simulink model "PID_Controller_xynew_2018"  (R2018b)
settings: Solver=ode4  StartTime=0.0  StopTime=50  FixedStep=0.01  RelTol=1e-5
InitFcn:
  | % load parameters of the default quadrotor
  | disp('Quadrotor parameters loaded by InitFcn')
  | mdl_quadrotor
undefined symbols (not defined in the file or in its folder): A, B, C, D, pwm, quad
libraries: vrlib x3, realtime_pacer_lib x2, simulink x1
(part 3 of 4)

== system PID_Controller_xynew_2018/Linear Controller/Position_controller/Subsystem1 ==
  a[0] : Inport
  a[1] : Inport  Port=2
  sin(yaw) : Inport  Port=3
  cos(yaw) : Inport  Port=4
  Gain : Gain  Gain=1/9.81
  Product : Product
  Product1 : Product
  Sum1 : Sum
  Pitch adjust : Outport
  wires:
  Sum1/1 -> Gain/1
  a[0]/1 -> Product/1
  Product/1 -> Sum1/1
  cos(yaw)/1 -> Product/2
  a[1]/1 -> Product1/1
  Product1/1 -> Sum1/2
  Gain/1 -> Pitch adjust/1
  sin(yaw)/1 -> Product1/2

== system PID_Controller_xynew_2018/Linear Controller/Position_controller/pitch controller ==
  x double dot : Inport
  y double dot : Inport  Port=2
  sin(yaw) : Inport  Port=3
  cos(yaw) : Inport  Port=4
  Fcn : Fcn  Expr=1/(u)
  Gain : Gain  Gain=1/9.81
  Product : Product
  Product1 : Product
  Product2 : Product
  Square : Math  Operator=square  SaturateOnIntegerOverflow=on
  Square1 : Math  Operator=square  SaturateOnIntegerOverflow=on
  Sum : Sum  Inputs=|-+
  Sum1 : Sum  Inputs=+-
  Roll adjust : Outport
  wires:
  Square/1 -> Sum/1
  Product1/1 -> Sum1/2
  sin(yaw)/1 -> Square1/1, Product/2
  Product2/1 -> Roll adjust/1
  cos(yaw)/1 -> Square/1, Product1/2
  Sum1/1 -> Gain/1
  x double dot/1 -> Product/1
  Product/1 -> Sum1/1
  Fcn/1 -> Product2/2
  Square1/1 -> Sum/2
  Gain/1 -> Product2/1
  Sum/1 -> Fcn/1
  y double dot/1 -> Product1/1

== system PID_Controller_xynew_2018/Linear Controller/Position_controller1/PID_Roll_Rate2 ==
  Setpoint : Inport
  Measured : Inport  Port=2
  Derivative : Derivative
  Integrator Limited : Integrator  LimitOutput=on  UpperSaturationLimit=0.1  LowerSaturationLimit=-0.1
  Kd : Gain  Gain=0  OutMin=[-200]  OutMax=[200]
  Ki : Gain  Gain=2  OutMin=[-200]  OutMax=[200]
  Kp : Gain  Gain=30  OutMin=[-200]  OutMax=[200]
  Scope : Scope
  Sum5 : Sum  Inputs=+++
  Sum6 : Sum  Inputs=+-|
  Adjust : Outport  VectorParamsAs1DForOutWhenUnconnected=on
  wires:
  Measured/1 -> Sum6/2  "measured"
  Setpoint/1 -> Sum6/1  "pid_desired"
  Ki/1 -> Sum5/2
  Sum5/1 -> Adjust/1
  Kp/1 -> Sum5/1
  Kd/1 -> Sum5/3
  Sum6/1 -> Derivative/1, Integrator Limited/1, Kp/1  "pid_error"
  Integrator Limited/1 -> Scope/1, Ki/1
  Derivative/1 -> Kd/1

== system PID_Controller_xynew_2018/Linear Controller/Position_controller1/PID_Roll_Rate3 ==
  Setpoint : Inport
  Measured : Inport  Port=2
  Derivative : Derivative
  Integrator Limited : Integrator  LimitOutput=on  UpperSaturationLimit=0.1  LowerSaturationLimit=-0.1
  Kd : Gain  Gain=0  OutMin=[-200]  OutMax=[200]
  Ki : Gain  Gain=-2  OutMin=[-200]  OutMax=[200]
  Kp : Gain  Gain=-30  OutMin=[-200]  OutMax=[200]
  Scope : Scope
  Sum5 : Sum  Inputs=+++
  Sum6 : Sum  Inputs=+-|
  Adjust : Outport  VectorParamsAs1DForOutWhenUnconnected=on
  wires:
  Derivative/1 -> Kd/1
  Integrator Limited/1 -> Ki/1, Scope/1
  Sum6/1 -> Kp/1, Integrator Limited/1, Derivative/1  "pid_error"
  Kd/1 -> Sum5/3
  Kp/1 -> Sum5/1
  Sum5/1 -> Adjust/1
  Ki/1 -> Sum5/2
  Setpoint/1 -> Sum6/1  "pid_desired"
  Measured/1 -> Sum6/2  "measured"

== system PID_Controller_xynew_2018/Linear Controller/Position_controller1/PID_X2 ==
  Setpoint : Inport
  Measured : Inport  Port=2
  1/dt : Gain  Gain=100  OutMin=[-200]  OutMax=[200]
  Kd : Gain  Gain=0  OutMin=[-200]  OutMax=[200]
  Ki : Gain  OutMin=[-200]  OutMax=[200]
  Kp : Gain  Gain=15  OutMin=[-200]  OutMax=[200]
  Memory : Memory
  Memory1 : Memory
  Saturation : Saturate  UpperLimit=0.1  LowerLimit=-0.1
  Scope1 : Scope
  Scope2 : Scope
  Sum1 : Sum  Inputs=|++
  Sum2 : Sum  Inputs=|+-
  Sum5 : Sum  Inputs=+++
  Sum6 : Sum  Inputs=+-|
  dt : Gain  Gain=1/100  OutMin=[-200]  OutMax=[200]
  Adjust : Outport  VectorParamsAs1DForOutWhenUnconnected=on
  wires:
  Measured/1 -> Sum6/2
  Saturation/1 -> Ki/1, Scope2/1
  Memory1/1 -> Sum1/2
  Sum1/1 -> Saturation/1, Scope1/1, Memory1/1  "pid_integ"
  Sum6/1 -> Kp/1, dt/1, Memory/1, Sum2/1  "pid_error"
  1/dt/1 -> Kd/1
  Sum2/1 -> 1/dt/1
  dt/1 -> Sum1/1
  Kd/1 -> Sum5/3
  Kp/1 -> Sum5/1
  Sum5/1 -> Adjust/1
  Ki/1 -> Sum5/2
  Memory/1 -> Sum2/2  "pid_prevError"
  Setpoint/1 -> Sum6/1  "pid_desired"

== system PID_Controller_xynew_2018/Linear Controller/Position_controller1/PID_Y2 ==
  Setpoint : Inport
  Measured : Inport  Port=2
  1/dt : Gain  Gain=100  OutMin=[-200]  OutMax=[200]
  Kd : Gain  Gain=0  OutMin=[-200]  OutMax=[200]
  Ki : Gain  Gain=-1  OutMin=[-200]  OutMax=[200]
  Kp : Gain  Gain=-15  OutMin=[-200]  OutMax=[200]
  Memory : Memory
  Memory1 : Memory
  Saturation : Saturate  UpperLimit=0.1  LowerLimit=-0.1
  Scope1 : Scope
  Scope2 : Scope
  Sum1 : Sum  Inputs=|++
  Sum2 : Sum  Inputs=|+-
  Sum5 : Sum  Inputs=+++
  Sum6 : Sum  Inputs=+-|
  dt : Gain  Gain=1/100  OutMin=[-200]  OutMax=[200]
  Adjust : Outport  VectorParamsAs1DForOutWhenUnconnected=on
  wires:
  Measured/1 -> Sum6/2
  Saturation/1 -> Ki/1, Scope2/1
  Memory1/1 -> Sum1/2
  Sum1/1 -> Saturation/1, Scope1/1, Memory1/1  "pid_integ"
  Sum6/1 -> Kp/1, dt/1, Memory/1, Sum2/1  "pid_error"
  1/dt/1 -> Kd/1
  Sum2/1 -> 1/dt/1
  dt/1 -> Sum1/1
  Kd/1 -> Sum5/3
  Kp/1 -> Sum5/1
  Sum5/1 -> Adjust/1
  Ki/1 -> Sum5/2
  Memory/1 -> Sum2/2  "pid_prevError"
  Setpoint/1 -> Sum6/1  "pid_desired"

== system PID_Controller_xynew_2018/Linear Controller/Rate_controller/PID_Pitch_Rate1 ==
  Setpoint : Inport
  Measured : Inport  Port=2
  1/dt : Gain  Gain=500  OutMin=[-200]  OutMax=[200]
  Kd : Gain  Gain=0  OutMin=[-200]  OutMax=[200]
  Ki : Gain  Gain=0  OutMin=[-200]  OutMax=[200]
  Kp : Gain  Gain=70  OutMin=[-200]  OutMax=[200]
  Memory : Memory
  Memory1 : Memory
  Saturation : Saturate  UpperLimit=33  LowerLimit=-33
  Sum1 : Sum  Inputs=|++
  Sum2 : Sum  Inputs=|+-
  Sum5 : Sum  Inputs=+++
  Sum6 : Sum  Inputs=+-|
  dt : Gain  Gain=1/500  OutMin=[-200]  OutMax=[200]
  Adjust : Outport  VectorParamsAs1DForOutWhenUnconnected=on
  wires:
  Saturation/1 -> Ki/1
  Memory1/1 -> Sum1/2
  Sum1/1 -> Memory1/1, Saturation/1  "pid_integ"
  Sum6/1 -> Kp/1, dt/1, Memory/1, Sum2/1  "pid_error"
  1/dt/1 -> Kd/1
  Sum2/1 -> 1/dt/1
  dt/1 -> Sum1/1
  Kd/1 -> Sum5/3
  Kp/1 -> Sum5/1
  Sum5/1 -> Adjust/1
  Ki/1 -> Sum5/2
  Memory/1 -> Sum2/2  "pid_prevError"
  Setpoint/1 -> Sum6/1  "pid_desired"
  Measured/1 -> Sum6/2  "measured"

== system PID_Controller_xynew_2018/Linear Controller/Rate_controller/PID_Pitch_Rate3 ==
  Setpoint : Inport
  Measured : Inport  Port=2
  1/dt : Gain  Gain=500  OutMin=[-200]  OutMax=[200]
  Kd : Gain  Gain=0  OutMin=[-200]  OutMax=[200]
  Ki : Gain  Gain=0  OutMin=[-200]  OutMax=[200]
  Kp : Gain  Gain=70  OutMin=[-200]  OutMax=[200]
  Memory : Memory
  Memory1 : Memory
  Saturation : Saturate  UpperLimit=33  LowerLimit=-33
  Sum1 : Sum  Inputs=|++
  Sum2 : Sum  Inputs=|+-
  Sum5 : Sum  Inputs=+++
  Sum6 : Sum  Inputs=+-|
  dt : Gain  Gain=1/500  OutMin=[-200]  OutMax=[200]
  Adjust : Outport  VectorParamsAs1DForOutWhenUnconnected=on
  wires:
  Measured/1 -> Sum6/2  "measured"
  Setpoint/1 -> Sum6/1  "pid_desired"
  Memory/1 -> Sum2/2  "pid_prevError"
  Ki/1 -> Sum5/2
  Sum5/1 -> Adjust/1
  Kp/1 -> Sum5/1
  Kd/1 -> Sum5/3
  dt/1 -> Sum1/1
  Sum2/1 -> 1/dt/1
  1/dt/1 -> Kd/1
  Sum6/1 -> Sum2/1, Memory/1, dt/1, Kp/1  "pid_error"
  Sum1/1 -> Saturation/1, Memory1/1  "pid_integ"
  Memory1/1 -> Sum1/2
  Saturation/1 -> Ki/1

== system PID_Controller_xynew_2018/Linear Controller/Rate_controller/PID_Roll_Rate1 ==
  Setpoint : Inport
  Measured : Inport  Port=2
  Derivative : Derivative
  Integrator Limited : Integrator  LimitOutput=on  UpperSaturationLimit=1000  LowerSaturationLimit=-1000
  Kd : Gain  Gain=0  OutMin=[-200]  OutMax=[200]
  Ki : Gain  Gain=0  OutMin=[-200]  OutMax=[200]
  Kp : Gain  Gain=70  OutMin=[-200]  OutMax=[200]
  Scope : Scope
  Sum5 : Sum  Inputs=+++
  Sum6 : Sum  Inputs=+-|
  Adjust : Outport  VectorParamsAs1DForOutWhenUnconnected=on
  wires:
  Measured/1 -> Sum6/2  "measured"
  Setpoint/1 -> Sum6/1  "pid_desired"
  Ki/1 -> Sum5/2
  Sum5/1 -> Adjust/1
  Kp/1 -> Sum5/1
  Kd/1 -> Sum5/3
  Sum6/1 -> Derivative/1, Integrator Limited/1, Kp/1  "pid_error"
  Integrator Limited/1 -> Scope/1, Ki/1
  Derivative/1 -> Kd/1

== system PID_Controller_xynew_2018/Linear Controller/Rate_controller/PID_Roll_Rate3 ==
  Setpoint : Inport
  Measured : Inport  Port=2
  Derivative : Derivative
  Integrator Limited : Integrator  LimitOutput=on  UpperSaturationLimit=1000  LowerSaturationLimit=-1000
  Kd : Gain  Gain=0  OutMin=[-200]  OutMax=[200]
  Ki : Gain  Gain=0  OutMin=[-200]  OutMax=[200]
  Kp : Gain  Gain=70  OutMin=[-200]  OutMax=[200]
  Scope : Scope
  Sum5 : Sum  Inputs=+++
  Sum6 : Sum  Inputs=+-|
  Adjust : Outport  VectorParamsAs1DForOutWhenUnconnected=on
  wires:
  Derivative/1 -> Kd/1
  Integrator Limited/1 -> Ki/1, Scope/1
  Sum6/1 -> Kp/1, Integrator Limited/1, Derivative/1  "pid_error"
  Kd/1 -> Sum5/3
  Kp/1 -> Sum5/1
  Sum5/1 -> Adjust/1
  Ki/1 -> Sum5/2
  Setpoint/1 -> Sum6/1  "pid_desired"
  Measured/1 -> Sum6/2  "measured"

== system PID_Controller_xynew_2018/Non linear controller/Altitude_controller/PID_Altitude ==
  Setpoint : Inport
  Measured : Inport  Port=2
  Derivative : Derivative
  Integrator Limited : Integrator  LimitOutput=on  UpperSaturationLimit=1000  LowerSaturationLimit=-1000
  Kd : Gain  Gain=9000  OutMin=[-200]  OutMax=[200]
  Ki : Gain  Gain=3500  OutMin=[-200]  OutMax=[200]
  Kp : Gain  Gain=11000  OutMin=[-200]  OutMax=[200]
  Sum5 : Sum  Inputs=+++
  Sum6 : Sum  Inputs=+-|
  Adjust : Outport  VectorParamsAs1DForOutWhenUnconnected=on
  wires:
  Derivative/1 -> Kd/1
  Integrator Limited/1 -> Ki/1
  Sum6/1 -> Kp/1, Integrator Limited/1, Derivative/1  "pid_error"
  Kd/1 -> Sum5/3
  Kp/1 -> Sum5/1
  Ki/1 -> Sum5/2
  Setpoint/1 -> Sum6/1  "pid_desired"
  Measured/1 -> Sum6/2  "measured"
  Sum5/1 -> Adjust/1

== system PID_Controller_xynew_2018/Non linear controller/Attitude_controller/PID_Pitch1 ==
  Setpoint : Inport
  Measured : Inport  Port=2
  1/dt : Gain  Gain=250  OutMin=[-200]  OutMax=[200]
  Kd : Gain  Gain=0  OutMin=[-200]  OutMax=[200]
  Ki : Gain  Gain=0  OutMin=[-200]  OutMax=[200]
  Kp : Gain  Gain=3.5  OutMin=[-200]  OutMax=[200]
  Memory : Memory
  Memory1 : Memory
  Saturation : Saturate  UpperLimit=20  LowerLimit=-20
  Sum1 : Sum  Inputs=|++
  Sum2 : Sum  Inputs=|+-
  Sum5 : Sum  Inputs=+++
  Sum6 : Sum  Inputs=+-|
  dt : Gain  Gain=1/250  OutMin=[-200]  OutMax=[200]
  Adjust : Outport  VectorParamsAs1DForOutWhenUnconnected=on
  wires:
  Saturation/1 -> Ki/1
  Memory1/1 -> Sum1/2
  Sum1/1 -> Saturation/1, Memory1/1  "pid_integ"
  Sum6/1 -> Kp/1, dt/1, Memory/1, Sum2/1  "pid_error"
  1/dt/1 -> Kd/1
  Sum2/1 -> 1/dt/1
  dt/1 -> Sum1/1
  Kd/1 -> Sum5/3
  Kp/1 -> Sum5/1
  Sum5/1 -> Adjust/1
  Ki/1 -> Sum5/2
  Memory/1 -> Sum2/2  "pid_prevError"
  Setpoint/1 -> Sum6/1  "pid_desired"
  Measured/1 -> Sum6/2  "measured"

== system PID_Controller_xynew_2018/Non linear controller/Attitude_controller/PID_Pitch3 ==
  Setpoint : Inport
  Measured : Inport  Port=2
  1/dt : Gain  Gain=250  OutMin=[-200]  OutMax=[200]
  Kd : Gain  Gain=0  OutMin=[-200]  OutMax=[200]
  Ki : Gain  Gain=0  OutMin=[-200]  OutMax=[200]
  Kp : Gain  Gain=3.5  OutMin=[-200]  OutMax=[200]
  Memory : Memory
  Memory1 : Memory
  Saturation : Saturate  UpperLimit=20  LowerLimit=-20
  Sum1 : Sum  Inputs=|++
  Sum2 : Sum  Inputs=|+-
  Sum5 : Sum  Inputs=+++
  Sum6 : Sum  Inputs=+-|
  dt : Gain  Gain=1/250  OutMin=[-200]  OutMax=[200]
  Adjust : Outport  VectorParamsAs1DForOutWhenUnconnected=on
  wires:
  Measured/1 -> Sum6/2  "measured"
  Setpoint/1 -> Sum6/1  "pid_desired"
  Memory/1 -> Sum2/2  "pid_prevError"
  Ki/1 -> Sum5/2
  Sum5/1 -> Adjust/1
  Kp/1 -> Sum5/1
  Kd/1 -> Sum5/3
  dt/1 -> Sum1/1
  Sum2/1 -> 1/dt/1
  1/dt/1 -> Kd/1
  Sum6/1 -> Sum2/1, Memory/1, dt/1, Kp/1  "pid_error"
  Sum1/1 -> Memory1/1, Saturation/1  "pid_integ"
  Memory1/1 -> Sum1/2
  Saturation/1 -> Ki/1

== system PID_Controller_xynew_2018/Non linear controller/Attitude_controller/PID_Pitch_Rate ==
  Setpoint : Inport
  Measured : Inport  Port=2
  Derivative : Derivative
  Integrator Limited : Integrator  LimitOutput=on  UpperSaturationLimit=20  LowerSaturationLimit=-20
  Kd : Gain  Gain=0  OutMin=[-200]  OutMax=[200]
  Ki : Gain  Gain=2  OutMin=[-200]  OutMax=[200]
  Kp : Gain  Gain=3.5  OutMin=[-200]  OutMax=[200]
  Sum5 : Sum  Inputs=+++
  Sum6 : Sum  Inputs=+-|
  Adjust : Outport  VectorParamsAs1DForOutWhenUnconnected=on
  wires:
  Derivative/1 -> Kd/1
  Integrator Limited/1 -> Ki/1
  Sum6/1 -> Kp/1, Integrator Limited/1, Derivative/1  "pid_error"
  Kd/1 -> Sum5/3
  Kp/1 -> Sum5/1
  Sum5/1 -> Adjust/1
  Ki/1 -> Sum5/2
  Setpoint/1 -> Sum6/1  "pid_desired"
  Measured/1 -> Sum6/2  "measured"

== system PID_Controller_xynew_2018/Non linear controller/Attitude_controller/PID_Roll_Rate ==
  Setpoint : Inport
  Measured : Inport  Port=2
  Derivative : Derivative
  Integrator Limited : Integrator  LimitOutput=on  UpperSaturationLimit=20  LowerSaturationLimit=-20
  Kd : Gain  Gain=0  OutMin=[-200]  OutMax=[200]
  Ki : Gain  Gain=2  OutMin=[-200]  OutMax=[200]
  Kp : Gain  Gain=3.5  OutMin=[-200]  OutMax=[200]
  Scope : Scope
  Sum5 : Sum  Inputs=+++
  Sum6 : Sum  Inputs=+-|
  Adjust : Outport  VectorParamsAs1DForOutWhenUnconnected=on
  wires:
  Measured/1 -> Sum6/2  "measured"
  Setpoint/1 -> Sum6/1  "pid_desired"
  Ki/1 -> Sum5/2
  Sum5/1 -> Adjust/1
  Kp/1 -> Sum5/1
  Kd/1 -> Sum5/3
  Sum6/1 -> Derivative/1, Integrator Limited/1, Kp/1  "pid_error"
  Integrator Limited/1 -> Scope/1, Ki/1
  Derivative/1 -> Kd/1

== system PID_Controller_xynew_2018/Non linear controller/Control_mixer/Configuration_+ ==
  Pitch : Inport
  Roll : Inport  Port=2
  Yaw : Inport  Port=3
  Tau : Inport  Port=4
  Sum{1,9..12} (5 alike) : Sum  Inputs=|++  SaturateOnIntegerOverflow=on  InputSameDT=on  OutDataTypeStr=Inherit: Same as first input
  Sum3 : Sum  Inputs=|--  SaturateOnIntegerOverflow=on  InputSameDT=on  OutDataTypeStr=Inherit: Same as first input
  Sum5 : Sum  Inputs=|-+  SaturateOnIntegerOverflow=on  InputSameDT=on  OutDataTypeStr=Inherit: Same as first input
  Sum7 : Sum  Inputs=|+-  SaturateOnIntegerOverflow=on  InputSameDT=on  OutDataTypeStr=Inherit: Same as first input
  W1 : Outport  VectorParamsAs1DForOutWhenUnconnected=on
  W2 : Outport  Port=2  VectorParamsAs1DForOutWhenUnconnected=on
  W3 : Outport  Port=3  VectorParamsAs1DForOutWhenUnconnected=on
  W4 : Outport  Port=4  VectorParamsAs1DForOutWhenUnconnected=on
  wires:
  Sum5/1 -> Sum11/1
  Yaw/1 -> Sum7/2, Sum5/2, Sum3/2, Sum1/2
  Tau/1 -> Sum11/2, Sum12/2, Sum10/2, Sum9/2
  Sum9/1 -> W1/1
  Pitch/1 -> Sum1/1, Sum5/1
  Roll/1 -> Sum3/1, Sum7/1
  Sum11/1 -> W3/1
  Sum12/1 -> W4/1
  Sum7/1 -> Sum12/1
  Sum10/1 -> W2/1
  Sum1/1 -> Sum9/1
  Sum3/1 -> Sum10/1

== system PID_Controller_xynew_2018/Non linear controller/Control_mixer/Configuration_X1 ==
  Pitch : Inport
  Roll : Inport  Port=2
  Yaw : Inport  Port=3
  Tau : Inport  Port=4
  Gain : Gain  Gain=0.5
  Gain1 : Gain  Gain=0.5
  Sum1 : Sum  Inputs=|+-+  SaturateOnIntegerOverflow=on  InputSameDT=on  OutDataTypeStr=Inherit: Same as first input
  Sum{9..12} (4 alike) : Sum  Inputs=|++  SaturateOnIntegerOverflow=on  InputSameDT=on  OutDataTypeStr=Inherit: Same as first input
  Sum3 : Sum  Inputs=|++-  SaturateOnIntegerOverflow=on  InputSameDT=on  OutDataTypeStr=Inherit: Same as first input
  Sum5 : Sum  Inputs=|+-+  SaturateOnIntegerOverflow=on  InputSameDT=on  OutDataTypeStr=Inherit: Same as first input
  Sum7 : Sum  Inputs=|---  SaturateOnIntegerOverflow=on  InputSameDT=on  OutDataTypeStr=Inherit: Same as first input
  W1 : Outport  VectorParamsAs1DForOutWhenUnconnected=on
  W2 : Outport  Port=2  VectorParamsAs1DForOutWhenUnconnected=on
  W3 : Outport  Port=3  VectorParamsAs1DForOutWhenUnconnected=on
  W4 : Outport  Port=4  VectorParamsAs1DForOutWhenUnconnected=on
  wires:
  Sum3/1 -> Sum11/1
  Yaw/1 -> Sum5/3, Sum3/3, Sum7/3, Sum1/3
  Tau/1 -> Sum11/2, Sum12/2, Sum10/2, Sum9/2
  Sum5/1 -> Sum12/1
  Sum7/1 -> Sum9/1
  Sum1/1 -> Sum10/1
  Roll/1 -> Gain1/1
  Pitch/1 -> Gain/1
  Gain/1 -> Sum7/1, Sum1/1, Sum5/2, Sum3/2
  Gain1/1 -> Sum7/2, Sum1/2, Sum5/1, Sum3/1
  Sum9/1 -> W1/1
  Sum10/1 -> W2/1
  Sum11/1 -> W3/1
  Sum12/1 -> W4/1

== system PID_Controller_xynew_2018/Non linear controller/Position_controller/PID_Roll_Rate1 ==
  Setpoint : Inport
  Measured : Inport  Port=2
  Derivative : Derivative
  Integrator Limited : Integrator  LimitOutput=on  UpperSaturationLimit=0.1  LowerSaturationLimit=-0.1
  Kd : Gain  Gain=0  OutMin=[-200]  OutMax=[200]
  Ki : Gain  Gain=2  OutMin=[-200]  OutMax=[200]
  Kp : Gain  Gain=30  OutMin=[-200]  OutMax=[200]
  Scope : Scope
  Sum5 : Sum  Inputs=+++
  Sum6 : Sum  Inputs=+-|
  Adjust : Outport  VectorParamsAs1DForOutWhenUnconnected=on
  wires:
  Measured/1 -> Sum6/2  "measured"
  Setpoint/1 -> Sum6/1  "pid_desired"
  Ki/1 -> Sum5/2
  Sum5/1 -> Adjust/1
  Kp/1 -> Sum5/1
  Kd/1 -> Sum5/3
  Sum6/1 -> Derivative/1, Integrator Limited/1, Kp/1  "pid_error"
  Integrator Limited/1 -> Scope/1, Ki/1
  Derivative/1 -> Kd/1

== system PID_Controller_xynew_2018/Non linear controller/Position_controller/PID_Roll_Rate2 ==
  "x_accel_cmd " : Inport
  y_accel_cmd : Inport  Port=2
  "yaw_traj " : Inport  Port=3
  "1/g " : Constant  Value=1/9.81
  Fcn : Fcn  Expr=sin(u)
  Fcn1 : Fcn  Expr=cos(u)
  Product : Product
  Product1 : Product
  Product2 : Product
  Sum : Sum  Inputs=|+-
  Adjust : Outport  VectorParamsAs1DForOutWhenUnconnected=on
  wires:
  "1/g "/1 -> Product/1
  "x_accel_cmd "/1 -> Product1/1
  "yaw_traj "/1 -> Fcn1/1, Fcn/1
  Fcn/1 -> Product1/2
  y_accel_cmd/1 -> Product2/1
  Fcn1/1 -> Product2/2
  Product1/1 -> Sum/1
  Product2/1 -> Sum/2
  Sum/1 -> Product/2
  Product/1 -> Adjust/1

== system PID_Controller_xynew_2018/Non linear controller/Position_controller/PID_Roll_Rate3 ==
  "x_accel_cmd " : Inport
  y_accel_cmd : Inport  Port=2
  "yaw_traj " : Inport  Port=3
  "1/g " : Constant  Value=1/9.81
  Fcn : Fcn  Expr=sin(u)
  Fcn1 : Fcn  Expr=cos(u)
  Product : Product
  Product1 : Product
  Product2 : Product
  Sum : Sum  Inputs=|+-
  Adjust : Outport  VectorParamsAs1DForOutWhenUnconnected=on
  wires:
  Product2/1 -> Sum/2
  Fcn1/1 -> Product2/2
  Sum/1 -> Product/2
  "x_accel_cmd "/1 -> Product1/1
  "1/g "/1 -> Product/1
  Product/1 -> Adjust/1
  y_accel_cmd/1 -> Product2/1
  Fcn/1 -> Product1/2
  Product1/1 -> Sum/1
  "yaw_traj "/1 -> Fcn1/1, Fcn/1

== system PID_Controller_xynew_2018/Non linear controller/Position_controller/PID_Roll_Rate4 ==
  Setpoint : Inport
  Measured : Inport  Port=2
  Derivative : Derivative
  Integrator Limited : Integrator  LimitOutput=on  UpperSaturationLimit=0.1  LowerSaturationLimit=-0.1
  Kd : Gain  Gain=0  OutMin=[-200]  OutMax=[200]
  Ki : Gain  Gain=-2  OutMin=[-200]  OutMax=[200]
  Kp : Gain  Gain=-30  OutMin=[-200]  OutMax=[200]
  Scope : Scope
  Sum5 : Sum  Inputs=+++
  Sum6 : Sum  Inputs=+-|
  Adjust : Outport  VectorParamsAs1DForOutWhenUnconnected=on
  wires:
  Derivative/1 -> Kd/1
  Integrator Limited/1 -> Ki/1, Scope/1
  Sum6/1 -> Kp/1, Integrator Limited/1, Derivative/1  "pid_error"
  Kd/1 -> Sum5/3
  Kp/1 -> Sum5/1
  Sum5/1 -> Adjust/1
  Ki/1 -> Sum5/2
  Setpoint/1 -> Sum6/1  "pid_desired"
  Measured/1 -> Sum6/2  "measured"

== system PID_Controller_xynew_2018/Non linear controller/Position_controller/PID_X2 ==
  Setpoint : Inport
  Measured : Inport  Port=2
  1/dt : Gain  Gain=100  OutMin=[-200]  OutMax=[200]
  Kd : Gain  Gain=0  OutMin=[-200]  OutMax=[200]
  Ki : Gain  OutMin=[-200]  OutMax=[200]
  Kp : Gain  Gain=15  OutMin=[-200]  OutMax=[200]
  Memory : Memory
  Memory1 : Memory
  Saturation : Saturate  UpperLimit=0.1  LowerLimit=-0.1
  Scope1 : Scope
  Scope2 : Scope
  Sum1 : Sum  Inputs=|++
  Sum2 : Sum  Inputs=|+-
  Sum5 : Sum  Inputs=+++
  Sum6 : Sum  Inputs=+-|
  dt : Gain  Gain=1/100  OutMin=[-200]  OutMax=[200]
  Adjust : Outport  VectorParamsAs1DForOutWhenUnconnected=on
  wires:
  Measured/1 -> Sum6/2
  Saturation/1 -> Ki/1, Scope2/1
  Memory1/1 -> Sum1/2
  Sum1/1 -> Saturation/1, Scope1/1, Memory1/1  "pid_integ"
  Sum6/1 -> Kp/1, dt/1, Memory/1, Sum2/1  "pid_error"
  1/dt/1 -> Kd/1
  Sum2/1 -> 1/dt/1
  dt/1 -> Sum1/1
  Kd/1 -> Sum5/3
  Kp/1 -> Sum5/1
  Sum5/1 -> Adjust/1
  Ki/1 -> Sum5/2
  Memory/1 -> Sum2/2  "pid_prevError"
  Setpoint/1 -> Sum6/1  "pid_desired"

== system PID_Controller_xynew_2018/Non linear controller/Position_controller/PID_Y2 ==
  Setpoint : Inport
  Measured : Inport  Port=2
  1/dt : Gain  Gain=100  OutMin=[-200]  OutMax=[200]
  Kd : Gain  Gain=0  OutMin=[-200]  OutMax=[200]
  Ki : Gain  Gain=-1  OutMin=[-200]  OutMax=[200]
  Kp : Gain  Gain=-15  OutMin=[-200]  OutMax=[200]
  Memory : Memory
  Memory1 : Memory
  Saturation : Saturate  UpperLimit=0.1  LowerLimit=-0.1
  Scope1 : Scope
  Scope2 : Scope
  Sum1 : Sum  Inputs=|++
  Sum2 : Sum  Inputs=|+-
  Sum5 : Sum  Inputs=+++
  Sum6 : Sum  Inputs=+-|
  dt : Gain  Gain=1/100  OutMin=[-200]  OutMax=[200]
  Adjust : Outport  VectorParamsAs1DForOutWhenUnconnected=on
  wires:
  Measured/1 -> Sum6/2
  Saturation/1 -> Ki/1, Scope2/1
  Memory1/1 -> Sum1/2
  Sum1/1 -> Saturation/1, Scope1/1, Memory1/1  "pid_integ"
  Sum6/1 -> Kp/1, dt/1, Memory/1, Sum2/1  "pid_error"
  1/dt/1 -> Kd/1
  Sum2/1 -> 1/dt/1
  dt/1 -> Sum1/1
  Kd/1 -> Sum5/3
  Kp/1 -> Sum5/1
  Sum5/1 -> Adjust/1
  Ki/1 -> Sum5/2
  Memory/1 -> Sum2/2  "pid_prevError"
  Setpoint/1 -> Sum6/1  "pid_desired"

== system PID_Controller_xynew_2018/Non linear controller/Position_controller/Roll controller ==
  x double dot : Inport
  y double dot : Inport  Port=2
  sin(yaw) : Inport  Port=3
  cos(yaw) : Inport  Port=4
  Fcn : Fcn  Expr=1/(u)
  Gain : Gain  Gain=1/9.81
  Product : Product
  Product1 : Product
  Product2 : Product
  Square : Math  Operator=square  SaturateOnIntegerOverflow=on
  Square1 : Math  Operator=square  SaturateOnIntegerOverflow=on
  Sum : Sum  Inputs=|+-
  Sum1 : Sum  Inputs=+-
  Roll adjust : Outport
  wires:
  x double dot/1 -> Product/1
  sin(yaw)/1 -> Product1/2, Square1/1
  Product/1 -> Sum1/1
  cos(yaw)/1 -> Product/2, Square/1
  y double dot/1 -> Product1/1
  Product1/1 -> Sum1/2
  Gain/1 -> Product2/1
  Sum1/1 -> Gain/1
  Square/1 -> Sum/1
  Square1/1 -> Sum/2
  Sum/1 -> Fcn/1
  Product2/1 -> Roll adjust/1
  Fcn/1 -> Product2/2

== system PID_Controller_xynew_2018/Non linear controller/Position_controller/Subsystem ==
  a[0] : Inport
  a[1] : Inport  Port=2
  sin(yaw) : Inport  Port=3
  cos(yaw) : Inport  Port=4
  Gain : Gain  Gain=1/9.81
  Product : Product
  Product1 : Product
  Sum1 : Sum  Inputs=+-
  Roll adjust : Outport
  wires:
  a[0]/1 -> Product/1
  sin(yaw)/1 -> Product/2
  Product/1 -> Sum1/1
  cos(yaw)/1 -> Product1/2
  a[1]/1 -> Product1/1
  Product1/1 -> Sum1/2
  Gain/1 -> Roll adjust/1
  Sum1/1 -> Gain/1

== system PID_Controller_xynew_2018/Non linear controller/Position_controller/Subsystem1 ==
  a[0] : Inport
  a[1] : Inport  Port=2
  sin(yaw) : Inport  Port=3
  cos(yaw) : Inport  Port=4
  Gain : Gain  Gain=1/9.81
  Product : Product
  Product1 : Product
  Sum1 : Sum
  Pitch adjust : Outport
  wires:
  Sum1/1 -> Gain/1
  a[0]/1 -> Product/1
  Product/1 -> Sum1/1
  cos(yaw)/1 -> Product/2
  a[1]/1 -> Product1/1
  Product1/1 -> Sum1/2
  Gain/1 -> Pitch adjust/1
  sin(yaw)/1 -> Product1/2

== system PID_Controller_xynew_2018/Non linear controller/Position_controller/pitch controller ==
  x double dot : Inport
  y double dot : Inport  Port=2
  sin(yaw) : Inport  Port=3
  cos(yaw) : Inport  Port=4
  Fcn : Fcn  Expr=1/(u)
  Gain : Gain  Gain=1/9.81
  Product : Product
  Product1 : Product
  Product2 : Product
  Square : Math  Operator=square  SaturateOnIntegerOverflow=on
  Square1 : Math  Operator=square  SaturateOnIntegerOverflow=on
  Sum : Sum  Inputs=|-+
  Sum1 : Sum  Inputs=+-
  Pitch adjust : Outport
  wires:
  Square/1 -> Sum/1
  Product1/1 -> Sum1/2
  sin(yaw)/1 -> Square1/1, Product/2
  Product2/1 -> Pitch adjust/1
  cos(yaw)/1 -> Square/1, Product1/2
  Sum1/1 -> Gain/1
  x double dot/1 -> Product/1
  Product/1 -> Sum1/1
  Fcn/1 -> Product2/2
  Square1/1 -> Sum/2
  Gain/1 -> Product2/1
  Sum/1 -> Fcn/1
  y double dot/1 -> Product1/1

== system PID_Controller_xynew_2018/Non linear controller/Position_controller1/PID_Roll_Rate2 ==
  Setpoint : Inport
  Measured : Inport  Port=2
  Derivative : Derivative
  Integrator Limited : Integrator  LimitOutput=on  UpperSaturationLimit=0.1  LowerSaturationLimit=-0.1
  Kd : Gain  Gain=0  OutMin=[-200]  OutMax=[200]
  Ki : Gain  Gain=2  OutMin=[-200]  OutMax=[200]
  Kp : Gain  Gain=30  OutMin=[-200]  OutMax=[200]
  Scope : Scope
  Sum5 : Sum  Inputs=+++
  Sum6 : Sum  Inputs=+-|
  Adjust : Outport  VectorParamsAs1DForOutWhenUnconnected=on
  wires:
  Measured/1 -> Sum6/2  "measured"
  Setpoint/1 -> Sum6/1  "pid_desired"
  Ki/1 -> Sum5/2
  Sum5/1 -> Adjust/1
  Kp/1 -> Sum5/1
  Kd/1 -> Sum5/3
  Sum6/1 -> Derivative/1, Integrator Limited/1, Kp/1  "pid_error"
  Integrator Limited/1 -> Scope/1, Ki/1
  Derivative/1 -> Kd/1

== system PID_Controller_xynew_2018/Non linear controller/Position_controller1/PID_Roll_Rate3 ==
  Setpoint : Inport
  Measured : Inport  Port=2
  Derivative : Derivative
  Integrator Limited : Integrator  LimitOutput=on  UpperSaturationLimit=0.1  LowerSaturationLimit=-0.1
  Kd : Gain  Gain=0  OutMin=[-200]  OutMax=[200]
  Ki : Gain  Gain=-2  OutMin=[-200]  OutMax=[200]
  Kp : Gain  Gain=-30  OutMin=[-200]  OutMax=[200]
  Scope : Scope
  Sum5 : Sum  Inputs=+++
  Sum6 : Sum  Inputs=+-|
  Adjust : Outport  VectorParamsAs1DForOutWhenUnconnected=on
  wires:
  Derivative/1 -> Kd/1
  Integrator Limited/1 -> Ki/1, Scope/1
  Sum6/1 -> Kp/1, Integrator Limited/1, Derivative/1  "pid_error"
  Kd/1 -> Sum5/3
  Kp/1 -> Sum5/1
  Sum5/1 -> Adjust/1
  Ki/1 -> Sum5/2
  Setpoint/1 -> Sum6/1  "pid_desired"
  Measured/1 -> Sum6/2  "measured"

== system PID_Controller_xynew_2018/Non linear controller/Position_controller1/PID_X2 ==
  Setpoint : Inport
  Measured : Inport  Port=2
  1/dt : Gain  Gain=100  OutMin=[-200]  OutMax=[200]
  Kd : Gain  Gain=0  OutMin=[-200]  OutMax=[200]
  Ki : Gain  OutMin=[-200]  OutMax=[200]
  Kp : Gain  Gain=15  OutMin=[-200]  OutMax=[200]
  Memory : Memory
  Memory1 : Memory
  Saturation : Saturate  UpperLimit=0.1  LowerLimit=-0.1
  Scope1 : Scope
  Scope2 : Scope
  Sum1 : Sum  Inputs=|++
  Sum2 : Sum  Inputs=|+-
  Sum5 : Sum  Inputs=+++
  Sum6 : Sum  Inputs=+-|
  dt : Gain  Gain=1/100  OutMin=[-200]  OutMax=[200]
  Adjust : Outport  VectorParamsAs1DForOutWhenUnconnected=on
  wires:
  Measured/1 -> Sum6/2
  Saturation/1 -> Ki/1, Scope2/1
  Memory1/1 -> Sum1/2
  Sum1/1 -> Saturation/1, Scope1/1, Memory1/1  "pid_integ"
  Sum6/1 -> Kp/1, dt/1, Memory/1, Sum2/1  "pid_error"
  1/dt/1 -> Kd/1
  Sum2/1 -> 1/dt/1
  dt/1 -> Sum1/1
  Kd/1 -> Sum5/3
  Kp/1 -> Sum5/1
  Sum5/1 -> Adjust/1
  Ki/1 -> Sum5/2
  Memory/1 -> Sum2/2  "pid_prevError"
  Setpoint/1 -> Sum6/1  "pid_desired"

== system PID_Controller_xynew_2018/Non linear controller/Position_controller1/PID_Y2 ==
  Setpoint : Inport
  Measured : Inport  Port=2
  1/dt : Gain  Gain=100  OutMin=[-200]  OutMax=[200]
  Kd : Gain  Gain=0  OutMin=[-200]  OutMax=[200]
  Ki : Gain  Gain=-1  OutMin=[-200]  OutMax=[200]
  Kp : Gain  Gain=-15  OutMin=[-200]  OutMax=[200]
  Memory : Memory
  Memory1 : Memory
  Saturation : Saturate  UpperLimit=0.1  LowerLimit=-0.1
  Scope1 : Scope
  Scope2 : Scope
  Sum1 : Sum  Inputs=|++
  Sum2 : Sum  Inputs=|+-
  Sum5 : Sum  Inputs=+++
  Sum6 : Sum  Inputs=+-|
  dt : Gain  Gain=1/100  OutMin=[-200]  OutMax=[200]
  Adjust : Outport  VectorParamsAs1DForOutWhenUnconnected=on
  wires:
  Measured/1 -> Sum6/2
  Saturation/1 -> Ki/1, Scope2/1
  Memory1/1 -> Sum1/2
  Sum1/1 -> Saturation/1, Scope1/1, Memory1/1  "pid_integ"
  Sum6/1 -> Kp/1, dt/1, Memory/1, Sum2/1  "pid_error"
  1/dt/1 -> Kd/1
  Sum2/1 -> 1/dt/1
  dt/1 -> Sum1/1
  Kd/1 -> Sum5/3
  Kp/1 -> Sum5/1
  Sum5/1 -> Adjust/1
  Ki/1 -> Sum5/2
  Memory/1 -> Sum2/2  "pid_prevError"
  Setpoint/1 -> Sum6/1  "pid_desired"

== system PID_Controller_xynew_2018/Non linear controller/Rate_controller/PID_Pitch_Rate1 ==
  Setpoint : Inport
  Measured : Inport  Port=2
  1/dt : Gain  Gain=500  OutMin=[-200]  OutMax=[200]
  Kd : Gain  Gain=0  OutMin=[-200]  OutMax=[200]
  Ki : Gain  Gain=0  OutMin=[-200]  OutMax=[200]
  Kp : Gain  Gain=70  OutMin=[-200]  OutMax=[200]
  Memory : Memory
  Memory1 : Memory
  Saturation : Saturate  UpperLimit=33  LowerLimit=-33
  Sum1 : Sum  Inputs=|++
  Sum2 : Sum  Inputs=|+-
  Sum5 : Sum  Inputs=+++
  Sum6 : Sum  Inputs=+-|
  dt : Gain  Gain=1/500  OutMin=[-200]  OutMax=[200]
  Adjust : Outport  VectorParamsAs1DForOutWhenUnconnected=on
  wires:
  Saturation/1 -> Ki/1
  Memory1/1 -> Sum1/2
  Sum1/1 -> Memory1/1, Saturation/1  "pid_integ"
  Sum6/1 -> Kp/1, dt/1, Memory/1, Sum2/1  "pid_error"
  1/dt/1 -> Kd/1
  Sum2/1 -> 1/dt/1
  dt/1 -> Sum1/1
  Kd/1 -> Sum5/3
  Kp/1 -> Sum5/1
  Sum5/1 -> Adjust/1
  Ki/1 -> Sum5/2
  Memory/1 -> Sum2/2  "pid_prevError"
  Setpoint/1 -> Sum6/1  "pid_desired"
  Measured/1 -> Sum6/2  "measured"

== system PID_Controller_xynew_2018/Non linear controller/Rate_controller/PID_Pitch_Rate3 ==
  Setpoint : Inport
  Measured : Inport  Port=2
  1/dt : Gain  Gain=500  OutMin=[-200]  OutMax=[200]
  Kd : Gain  Gain=0  OutMin=[-200]  OutMax=[200]
  Ki : Gain  Gain=0  OutMin=[-200]  OutMax=[200]
  Kp : Gain  Gain=70  OutMin=[-200]  OutMax=[200]
  Memory : Memory
  Memory1 : Memory
  Saturation : Saturate  UpperLimit=33  LowerLimit=-33
  Sum1 : Sum  Inputs=|++
  Sum2 : Sum  Inputs=|+-
  Sum5 : Sum  Inputs=+++
  Sum6 : Sum  Inputs=+-|
  dt : Gain  Gain=1/500  OutMin=[-200]  OutMax=[200]
  Adjust : Outport  VectorParamsAs1DForOutWhenUnconnected=on
  wires:
  Measured/1 -> Sum6/2  "measured"
  Setpoint/1 -> Sum6/1  "pid_desired"
  Memory/1 -> Sum2/2  "pid_prevError"
  Ki/1 -> Sum5/2
  Sum5/1 -> Adjust/1
  Kp/1 -> Sum5/1
  Kd/1 -> Sum5/3
  dt/1 -> Sum1/1
  Sum2/1 -> 1/dt/1
  1/dt/1 -> Kd/1
  Sum6/1 -> Sum2/1, Memory/1, dt/1, Kp/1  "pid_error"
  Sum1/1 -> Saturation/1, Memory1/1  "pid_integ"
  Memory1/1 -> Sum1/2
  Saturation/1 -> Ki/1

== system PID_Controller_xynew_2018/Non linear controller/Rate_controller/PID_Roll_Rate1 ==
  Setpoint : Inport
  Measured : Inport  Port=2
  Derivative : Derivative
  Integrator Limited : Integrator  LimitOutput=on  UpperSaturationLimit=1000  LowerSaturationLimit=-1000
  Kd : Gain  Gain=0  OutMin=[-200]  OutMax=[200]
  Ki : Gain  Gain=0  OutMin=[-200]  OutMax=[200]
  Kp : Gain  Gain=70  OutMin=[-200]  OutMax=[200]
  Scope : Scope
  Sum5 : Sum  Inputs=+++
  Sum6 : Sum  Inputs=+-|
  Adjust : Outport  VectorParamsAs1DForOutWhenUnconnected=on
  wires:
  Measured/1 -> Sum6/2  "measured"
  Setpoint/1 -> Sum6/1  "pid_desired"
  Ki/1 -> Sum5/2
  Sum5/1 -> Adjust/1
  Kp/1 -> Sum5/1
  Kd/1 -> Sum5/3
  Sum6/1 -> Derivative/1, Integrator Limited/1, Kp/1  "pid_error"
  Integrator Limited/1 -> Scope/1, Ki/1
  Derivative/1 -> Kd/1

== system PID_Controller_xynew_2018/Non linear controller/Rate_controller/PID_Roll_Rate3 ==
  Setpoint : Inport
  Measured : Inport  Port=2
  Derivative : Derivative
  Integrator Limited : Integrator  LimitOutput=on  UpperSaturationLimit=1000  LowerSaturationLimit=-1000
  Kd : Gain  Gain=0  OutMin=[-200]  OutMax=[200]
  Ki : Gain  Gain=0  OutMin=[-200]  OutMax=[200]
  Kp : Gain  Gain=70  OutMin=[-200]  OutMax=[200]
  Scope : Scope
  Sum5 : Sum  Inputs=+++
  Sum6 : Sum  Inputs=+-|
  Adjust : Outport  VectorParamsAs1DForOutWhenUnconnected=on
  wires:
  Derivative/1 -> Kd/1
  Integrator Limited/1 -> Ki/1, Scope/1
  Sum6/1 -> Kp/1, Integrator Limited/1, Derivative/1  "pid_error"
  Kd/1 -> Sum5/3
  Kp/1 -> Sum5/1
  Sum5/1 -> Adjust/1
  Ki/1 -> Sum5/2
  Setpoint/1 -> Sum6/1  "pid_desired"
  Measured/1 -> Sum6/2  "measured"

== system PID_Controller_xynew_2018/old linear backup/Altitude_controller/PID_Altitude ==
  Setpoint : Inport
  Measured : Inport  Port=2
  Derivative : Derivative
  Integrator Limited : Integrator  LimitOutput=on  UpperSaturationLimit=1000  LowerSaturationLimit=-1000
  Kd : Gain  Gain=9000  OutMin=[-200]  OutMax=[200]
  Ki : Gain  Gain=3500  OutMin=[-200]  OutMax=[200]
  Kp : Gain  Gain=11000  OutMin=[-200]  OutMax=[200]
  Sum5 : Sum  Inputs=+++
  Sum6 : Sum  Inputs=+-|
  Adjust : Outport  VectorParamsAs1DForOutWhenUnconnected=on
  wires:
  Derivative/1 -> Kd/1
  Integrator Limited/1 -> Ki/1
  Sum6/1 -> Kp/1, Integrator Limited/1, Derivative/1  "pid_error"
  Kd/1 -> Sum5/3
  Kp/1 -> Sum5/1
  Ki/1 -> Sum5/2
  Setpoint/1 -> Sum6/1  "pid_desired"
  Measured/1 -> Sum6/2  "measured"
  Sum5/1 -> Adjust/1

== system PID_Controller_xynew_2018/old linear backup/Attitude_controller/PID_Pitch1 ==
  Setpoint : Inport
  Measured : Inport  Port=2
  1/dt : Gain  Gain=250  OutMin=[-200]  OutMax=[200]
  Kd : Gain  Gain=0  OutMin=[-200]  OutMax=[200]
  Ki : Gain  Gain=0  OutMin=[-200]  OutMax=[200]
  Kp : Gain  Gain=3.5  OutMin=[-200]  OutMax=[200]
  Memory : Memory
  Memory1 : Memory
  Saturation : Saturate  UpperLimit=20  LowerLimit=-20
  Sum1 : Sum  Inputs=|++
  Sum2 : Sum  Inputs=|+-
  Sum5 : Sum  Inputs=+++
  Sum6 : Sum  Inputs=+-|
  dt : Gain  Gain=1/250  OutMin=[-200]  OutMax=[200]
  Adjust : Outport  VectorParamsAs1DForOutWhenUnconnected=on
  wires:
  Saturation/1 -> Ki/1
  Memory1/1 -> Sum1/2
  Sum1/1 -> Saturation/1, Memory1/1  "pid_integ"
  Sum6/1 -> Kp/1, dt/1, Memory/1, Sum2/1  "pid_error"
  1/dt/1 -> Kd/1
  Sum2/1 -> 1/dt/1
  dt/1 -> Sum1/1
  Kd/1 -> Sum5/3
  Kp/1 -> Sum5/1
  Sum5/1 -> Adjust/1
  Ki/1 -> Sum5/2
  Memory/1 -> Sum2/2  "pid_prevError"
  Setpoint/1 -> Sum6/1  "pid_desired"
  Measured/1 -> Sum6/2  "measured"

== system PID_Controller_xynew_2018/old linear backup/Attitude_controller/PID_Pitch3 ==
  Setpoint : Inport
  Measured : Inport  Port=2
  1/dt : Gain  Gain=250  OutMin=[-200]  OutMax=[200]
  Kd : Gain  Gain=0  OutMin=[-200]  OutMax=[200]
  Ki : Gain  Gain=0  OutMin=[-200]  OutMax=[200]
  Kp : Gain  Gain=3.5  OutMin=[-200]  OutMax=[200]
  Memory : Memory
  Memory1 : Memory
  Saturation : Saturate  UpperLimit=20  LowerLimit=-20
  Sum1 : Sum  Inputs=|++
  Sum2 : Sum  Inputs=|+-
  Sum5 : Sum  Inputs=+++
  Sum6 : Sum  Inputs=+-|
  dt : Gain  Gain=1/250  OutMin=[-200]  OutMax=[200]
  Adjust : Outport  VectorParamsAs1DForOutWhenUnconnected=on
  wires:
  Measured/1 -> Sum6/2  "measured"
  Setpoint/1 -> Sum6/1  "pid_desired"
  Memory/1 -> Sum2/2  "pid_prevError"
  Ki/1 -> Sum5/2
  Sum5/1 -> Adjust/1
  Kp/1 -> Sum5/1
  Kd/1 -> Sum5/3
  dt/1 -> Sum1/1
  Sum2/1 -> 1/dt/1
  1/dt/1 -> Kd/1
  Sum6/1 -> Sum2/1, Memory/1, dt/1, Kp/1  "pid_error"
  Sum1/1 -> Memory1/1, Saturation/1  "pid_integ"
  Memory1/1 -> Sum1/2
  Saturation/1 -> Ki/1

== system PID_Controller_xynew_2018/old linear backup/Attitude_controller/PID_Roll_Rate1 ==
  Setpoint : Inport
  Measured : Inport  Port=2
  Derivative : Derivative
  Integrator Limited : Integrator  LimitOutput=on  UpperSaturationLimit=20  LowerSaturationLimit=-20
  Kd : Gain  Gain=0  OutMin=[-200]  OutMax=[200]
  Ki : Gain  Gain=2  OutMin=[-200]  OutMax=[200]
  Kp : Gain  Gain=3.5  OutMin=[-200]  OutMax=[200]
  Scope : Scope
  Sum5 : Sum  Inputs=+++
  Sum6 : Sum  Inputs=+-|
  Adjust : Outport  VectorParamsAs1DForOutWhenUnconnected=on
  wires:
  Measured/1 -> Sum6/2  "measured"
  Setpoint/1 -> Sum6/1  "pid_desired"
  Ki/1 -> Sum5/2
  Sum5/1 -> Adjust/1
  Kp/1 -> Sum5/1
  Kd/1 -> Sum5/3
  Sum6/1 -> Derivative/1, Integrator Limited/1, Kp/1  "pid_error"
  Integrator Limited/1 -> Scope/1, Ki/1
  Derivative/1 -> Kd/1

== system PID_Controller_xynew_2018/old linear backup/Attitude_controller/PID_Roll_Rate2 ==
  Setpoint : Inport
  Measured : Inport  Port=2
  Derivative : Derivative
  Integrator Limited : Integrator  LimitOutput=on  UpperSaturationLimit=20  LowerSaturationLimit=-20
  Kd : Gain  Gain=0  OutMin=[-200]  OutMax=[200]
  Ki : Gain  Gain=2  OutMin=[-200]  OutMax=[200]
  Kp : Gain  Gain=3.5  OutMin=[-200]  OutMax=[200]
  Scope : Scope
  Sum5 : Sum  Inputs=+++
  Sum6 : Sum  Inputs=+-|
  Adjust : Outport  VectorParamsAs1DForOutWhenUnconnected=on
  wires:
  Derivative/1 -> Kd/1
  Integrator Limited/1 -> Ki/1, Scope/1
  Sum6/1 -> Kp/1, Integrator Limited/1, Derivative/1  "pid_error"
  Kd/1 -> Sum5/3
  Kp/1 -> Sum5/1
  Sum5/1 -> Adjust/1
  Ki/1 -> Sum5/2
  Setpoint/1 -> Sum6/1  "pid_desired"
  Measured/1 -> Sum6/2  "measured"

== system PID_Controller_xynew_2018/old linear backup/Control_mixer/Configuration_+ ==
  Pitch : Inport
  Roll : Inport  Port=2
  Yaw : Inport  Port=3
  Tau : Inport  Port=4
  Sum{1,9..12} (5 alike) : Sum  Inputs=|++  SaturateOnIntegerOverflow=on  InputSameDT=on  OutDataTypeStr=Inherit: Same as first input
  Sum3 : Sum  Inputs=|--  SaturateOnIntegerOverflow=on  InputSameDT=on  OutDataTypeStr=Inherit: Same as first input
  Sum5 : Sum  Inputs=|-+  SaturateOnIntegerOverflow=on  InputSameDT=on  OutDataTypeStr=Inherit: Same as first input
  Sum7 : Sum  Inputs=|+-  SaturateOnIntegerOverflow=on  InputSameDT=on  OutDataTypeStr=Inherit: Same as first input
  W1 : Outport  VectorParamsAs1DForOutWhenUnconnected=on
  W2 : Outport  Port=2  VectorParamsAs1DForOutWhenUnconnected=on
  W3 : Outport  Port=3  VectorParamsAs1DForOutWhenUnconnected=on
  W4 : Outport  Port=4  VectorParamsAs1DForOutWhenUnconnected=on
  wires:
  Sum5/1 -> Sum11/1
  Yaw/1 -> Sum7/2, Sum5/2, Sum3/2, Sum1/2
  Tau/1 -> Sum11/2, Sum12/2, Sum10/2, Sum9/2
  Sum9/1 -> W1/1
  Pitch/1 -> Sum1/1, Sum5/1
  Roll/1 -> Sum3/1, Sum7/1
  Sum11/1 -> W3/1
  Sum12/1 -> W4/1
  Sum7/1 -> Sum12/1
  Sum10/1 -> W2/1
  Sum1/1 -> Sum9/1
  Sum3/1 -> Sum10/1

== system PID_Controller_xynew_2018/old linear backup/Control_mixer/Configuration_X1 ==
  Pitch : Inport
  Roll : Inport  Port=2
  Yaw : Inport  Port=3
  Tau : Inport  Port=4
  Gain : Gain  Gain=0.5
  Gain1 : Gain  Gain=0.5
  Sum1 : Sum  Inputs=|+-+  SaturateOnIntegerOverflow=on  InputSameDT=on  OutDataTypeStr=Inherit: Same as first input
  Sum{9..12} (4 alike) : Sum  Inputs=|++  SaturateOnIntegerOverflow=on  InputSameDT=on  OutDataTypeStr=Inherit: Same as first input
  Sum3 : Sum  Inputs=|++-  SaturateOnIntegerOverflow=on  InputSameDT=on  OutDataTypeStr=Inherit: Same as first input
  Sum5 : Sum  Inputs=|+-+  SaturateOnIntegerOverflow=on  InputSameDT=on  OutDataTypeStr=Inherit: Same as first input
  Sum7 : Sum  Inputs=|---  SaturateOnIntegerOverflow=on  InputSameDT=on  OutDataTypeStr=Inherit: Same as first input
  W1 : Outport  VectorParamsAs1DForOutWhenUnconnected=on
  W2 : Outport  Port=2  VectorParamsAs1DForOutWhenUnconnected=on
  W3 : Outport  Port=3  VectorParamsAs1DForOutWhenUnconnected=on
  W4 : Outport  Port=4  VectorParamsAs1DForOutWhenUnconnected=on
  wires:
  Sum3/1 -> Sum11/1
  Yaw/1 -> Sum5/3, Sum3/3, Sum7/3, Sum1/3
  Tau/1 -> Sum11/2, Sum12/2, Sum10/2, Sum9/2
  Sum5/1 -> Sum12/1
  Sum7/1 -> Sum9/1
  Sum1/1 -> Sum10/1
  Roll/1 -> Gain1/1
  Pitch/1 -> Gain/1
  Gain/1 -> Sum7/1, Sum1/1, Sum5/2, Sum3/2
  Gain1/1 -> Sum7/2, Sum1/2, Sum5/1, Sum3/1
  Sum9/1 -> W1/1
  Sum10/1 -> W2/1
  Sum11/1 -> W3/1
  Sum12/1 -> W4/1

== system PID_Controller_xynew_2018/old linear backup/Position_controller/PID_Roll_Rate1 ==
  Setpoint : Inport
  Measured : Inport  Port=2
  Derivative : Derivative
  Integrator Limited : Integrator  LimitOutput=on  UpperSaturationLimit=0.1  LowerSaturationLimit=-0.1
  Kd : Gain  Gain=0  OutMin=[-200]  OutMax=[200]
  Ki : Gain  Gain=2  OutMin=[-200]  OutMax=[200]
  Kp : Gain  Gain=30  OutMin=[-200]  OutMax=[200]
  Scope : Scope
  Sum5 : Sum  Inputs=+++
  Sum6 : Sum  Inputs=+-|
  Adjust : Outport  VectorParamsAs1DForOutWhenUnconnected=on
  wires:
  Measured/1 -> Sum6/2  "measured"
  Setpoint/1 -> Sum6/1  "pid_desired"
  Ki/1 -> Sum5/2
  Sum5/1 -> Adjust/1
  Kp/1 -> Sum5/1
  Kd/1 -> Sum5/3
  Sum6/1 -> Derivative/1, Integrator Limited/1, Kp/1  "pid_error"
  Integrator Limited/1 -> Scope/1, Ki/1
  Derivative/1 -> Kd/1

== system PID_Controller_xynew_2018/old linear backup/Position_controller/PID_Roll_Rate2 ==
  "x_accel_cmd " : Inport
  y_accel_cmd : Inport  Port=2
  "yaw_traj " : Inport  Port=3
  "1/g " : Constant  Value=1/9.81
  Fcn : Fcn  Expr=sin(u)
  Fcn1 : Fcn  Expr=cos(u)
  Product : Product
  Product1 : Product
  Product2 : Product
  Sum : Sum  Inputs=|+-
  Adjust : Outport  VectorParamsAs1DForOutWhenUnconnected=on
  wires:
  "1/g "/1 -> Product/1
  "x_accel_cmd "/1 -> Product1/1
  "yaw_traj "/1 -> Fcn1/1, Fcn/1
  Fcn/1 -> Product1/2
  y_accel_cmd/1 -> Product2/1
  Fcn1/1 -> Product2/2
  Product1/1 -> Sum/1
  Product2/1 -> Sum/2
  Sum/1 -> Product/2
  Product/1 -> Adjust/1

== system PID_Controller_xynew_2018/old linear backup/Position_controller/PID_Roll_Rate3 ==
  "x_accel_cmd " : Inport
  y_accel_cmd : Inport  Port=2
  "yaw_traj " : Inport  Port=3
  "1/g " : Constant  Value=1/9.81
  Fcn : Fcn  Expr=sin(u)
  Fcn1 : Fcn  Expr=cos(u)
  Product : Product
  Product1 : Product
  Product2 : Product
  Sum : Sum  Inputs=|+-
  Adjust : Outport  VectorParamsAs1DForOutWhenUnconnected=on
  wires:
  Product2/1 -> Sum/2
  Fcn1/1 -> Product2/2
  Sum/1 -> Product/2
  "x_accel_cmd "/1 -> Product1/1
  "1/g "/1 -> Product/1
  Product/1 -> Adjust/1
  y_accel_cmd/1 -> Product2/1
  Fcn/1 -> Product1/2
  Product1/1 -> Sum/1
  "yaw_traj "/1 -> Fcn1/1, Fcn/1

== system PID_Controller_xynew_2018/old linear backup/Position_controller/PID_Roll_Rate4 ==
  Setpoint : Inport
  Measured : Inport  Port=2
  Derivative : Derivative
  Integrator Limited : Integrator  LimitOutput=on  UpperSaturationLimit=0.1  LowerSaturationLimit=-0.1
  Kd : Gain  Gain=0  OutMin=[-200]  OutMax=[200]
  Ki : Gain  Gain=-2  OutMin=[-200]  OutMax=[200]
  Kp : Gain  Gain=-30  OutMin=[-200]  OutMax=[200]
  Scope : Scope
  Sum5 : Sum  Inputs=+++
  Sum6 : Sum  Inputs=+-|
  Adjust : Outport  VectorParamsAs1DForOutWhenUnconnected=on
  wires:
  Derivative/1 -> Kd/1
  Integrator Limited/1 -> Ki/1, Scope/1
  Sum6/1 -> Kp/1, Integrator Limited/1, Derivative/1  "pid_error"
  Kd/1 -> Sum5/3
  Kp/1 -> Sum5/1
  Sum5/1 -> Adjust/1
  Ki/1 -> Sum5/2
  Setpoint/1 -> Sum6/1  "pid_desired"
  Measured/1 -> Sum6/2  "measured"

== system PID_Controller_xynew_2018/old linear backup/Position_controller/PID_X2 ==
  Setpoint : Inport
  Measured : Inport  Port=2
  1/dt : Gain  Gain=100  OutMin=[-200]  OutMax=[200]
  Kd : Gain  Gain=0  OutMin=[-200]  OutMax=[200]
  Ki : Gain  OutMin=[-200]  OutMax=[200]
  Kp : Gain  Gain=15  OutMin=[-200]  OutMax=[200]
  Memory : Memory
  Memory1 : Memory
  Saturation : Saturate  UpperLimit=0.1  LowerLimit=-0.1
  Scope1 : Scope
  Scope2 : Scope
  Sum1 : Sum  Inputs=|++
  Sum2 : Sum  Inputs=|+-
  Sum5 : Sum  Inputs=+++
  Sum6 : Sum  Inputs=+-|
  dt : Gain  Gain=1/100  OutMin=[-200]  OutMax=[200]
  Adjust : Outport  VectorParamsAs1DForOutWhenUnconnected=on
  wires:
  Measured/1 -> Sum6/2
  Saturation/1 -> Ki/1, Scope2/1
  Memory1/1 -> Sum1/2
  Sum1/1 -> Saturation/1, Scope1/1, Memory1/1  "pid_integ"
  Sum6/1 -> Kp/1, dt/1, Memory/1, Sum2/1  "pid_error"
  1/dt/1 -> Kd/1
  Sum2/1 -> 1/dt/1
  dt/1 -> Sum1/1
  Kd/1 -> Sum5/3
  Kp/1 -> Sum5/1
  Sum5/1 -> Adjust/1
  Ki/1 -> Sum5/2
  Memory/1 -> Sum2/2  "pid_prevError"
  Setpoint/1 -> Sum6/1  "pid_desired"

== system PID_Controller_xynew_2018/old linear backup/Position_controller/PID_Y2 ==
  Setpoint : Inport
  Measured : Inport  Port=2
  1/dt : Gain  Gain=100  OutMin=[-200]  OutMax=[200]
  Kd : Gain  Gain=0  OutMin=[-200]  OutMax=[200]
  Ki : Gain  Gain=-1  OutMin=[-200]  OutMax=[200]
  Kp : Gain  Gain=-15  OutMin=[-200]  OutMax=[200]
  Memory : Memory
  Memory1 : Memory
  Saturation : Saturate  UpperLimit=0.1  LowerLimit=-0.1
  Scope1 : Scope
  Scope2 : Scope
  Sum1 : Sum  Inputs=|++
  Sum2 : Sum  Inputs=|+-
  Sum5 : Sum  Inputs=+++
  Sum6 : Sum  Inputs=+-|
  dt : Gain  Gain=1/100  OutMin=[-200]  OutMax=[200]
  Adjust : Outport  VectorParamsAs1DForOutWhenUnconnected=on
  wires:
  Measured/1 -> Sum6/2
  Saturation/1 -> Ki/1, Scope2/1
  Memory1/1 -> Sum1/2
  Sum1/1 -> Saturation/1, Scope1/1, Memory1/1  "pid_integ"
  Sum6/1 -> Kp/1, dt/1, Memory/1, Sum2/1  "pid_error"
  1/dt/1 -> Kd/1
  Sum2/1 -> 1/dt/1
  dt/1 -> Sum1/1
  Kd/1 -> Sum5/3
  Kp/1 -> Sum5/1
  Sum5/1 -> Adjust/1
  Ki/1 -> Sum5/2
  Memory/1 -> Sum2/2  "pid_prevError"
  Setpoint/1 -> Sum6/1  "pid_desired"

== system PID_Controller_xynew_2018/old linear backup/Position_controller/Subsystem ==
  a[0] : Inport
  a[1] : Inport  Port=2
  sin(yaw) : Inport  Port=3
  cos(yaw) : Inport  Port=4
  Gain : Gain  Gain=-1/9.81
  Product : Product
  Product1 : Product
  Sum1 : Sum  Inputs=+-
  Pitch adjust : Outport
  wires:
  Sum1/1 -> Gain/1  "Accel cmd"
  a[0]/1 -> Product/1
  sin(yaw)/1 -> Product/2
  Product/1 -> Sum1/1
  cos(yaw)/1 -> Product1/2
  a[1]/1 -> Product1/1
  Product1/1 -> Sum1/2
  Gain/1 -> Pitch adjust/1

== system PID_Controller_xynew_2018/old linear backup/Position_controller/Subsystem1 ==
  a[0] : Inport
  a[1] : Inport  Port=2
  sin(yaw) : Inport  Port=3
  cos(yaw) : Inport  Port=4
  Gain : Gain  Gain=-1/9.81
  Product : Product
  Product1 : Product
  Sum1 : Sum
  Pitch adjust : Outport
  wires:
  Sum1/1 -> Gain/1
  a[0]/1 -> Product/1
  Product/1 -> Sum1/1
  cos(yaw)/1 -> Product/2
  a[1]/1 -> Product1/1
  Product1/1 -> Sum1/2
  Gain/1 -> Pitch adjust/1
  sin(yaw)/1 -> Product1/2

== system PID_Controller_xynew_2018/old linear backup/Position_controller1/PID_Roll_Rate2 ==
  Setpoint : Inport
  Measured : Inport  Port=2
  Derivative : Derivative
  Integrator Limited : Integrator  LimitOutput=on  UpperSaturationLimit=0.1  LowerSaturationLimit=-0.1
  Kd : Gain  Gain=0  OutMin=[-200]  OutMax=[200]
  Ki : Gain  Gain=2  OutMin=[-200]  OutMax=[200]
  Kp : Gain  Gain=30  OutMin=[-200]  OutMax=[200]
  Scope : Scope
  Sum5 : Sum  Inputs=+++
  Sum6 : Sum  Inputs=+-|
  Adjust : Outport  VectorParamsAs1DForOutWhenUnconnected=on
  wires:
  Measured/1 -> Sum6/2  "measured"
  Setpoint/1 -> Sum6/1  "pid_desired"
  Ki/1 -> Sum5/2
  Sum5/1 -> Adjust/1
  Kp/1 -> Sum5/1
  Kd/1 -> Sum5/3
  Sum6/1 -> Derivative/1, Integrator Limited/1, Kp/1  "pid_error"
  Integrator Limited/1 -> Scope/1, Ki/1
  Derivative/1 -> Kd/1

== system PID_Controller_xynew_2018/old linear backup/Position_controller1/PID_Roll_Rate3 ==
  Setpoint : Inport
  Measured : Inport  Port=2
  Derivative : Derivative
  Integrator Limited : Integrator  LimitOutput=on  UpperSaturationLimit=0.1  LowerSaturationLimit=-0.1
  Kd : Gain  Gain=0  OutMin=[-200]  OutMax=[200]
  Ki : Gain  Gain=-2  OutMin=[-200]  OutMax=[200]
  Kp : Gain  Gain=-30  OutMin=[-200]  OutMax=[200]
  Scope : Scope
  Sum5 : Sum  Inputs=+++
  Sum6 : Sum  Inputs=+-|
  Adjust : Outport  VectorParamsAs1DForOutWhenUnconnected=on
  wires:
  Derivative/1 -> Kd/1
  Integrator Limited/1 -> Ki/1, Scope/1
  Sum6/1 -> Kp/1, Integrator Limited/1, Derivative/1  "pid_error"
  Kd/1 -> Sum5/3
  Kp/1 -> Sum5/1
  Sum5/1 -> Adjust/1
  Ki/1 -> Sum5/2
  Setpoint/1 -> Sum6/1  "pid_desired"
  Measured/1 -> Sum6/2  "measured"

== system PID_Controller_xynew_2018/old linear backup/Position_controller1/PID_X2 ==
  Setpoint : Inport
  Measured : Inport  Port=2
  1/dt : Gain  Gain=100  OutMin=[-200]  OutMax=[200]
  Kd : Gain  Gain=0  OutMin=[-200]  OutMax=[200]
  Ki : Gain  OutMin=[-200]  OutMax=[200]
  Kp : Gain  Gain=15  OutMin=[-200]  OutMax=[200]
  Memory : Memory
  Memory1 : Memory
  Saturation : Saturate  UpperLimit=0.1  LowerLimit=-0.1
  Scope1 : Scope
  Scope2 : Scope
  Sum1 : Sum  Inputs=|++
  Sum2 : Sum  Inputs=|+-
  Sum5 : Sum  Inputs=+++
  Sum6 : Sum  Inputs=+-|
  dt : Gain  Gain=1/100  OutMin=[-200]  OutMax=[200]
  Adjust : Outport  VectorParamsAs1DForOutWhenUnconnected=on
  wires:
  Measured/1 -> Sum6/2
  Saturation/1 -> Ki/1, Scope2/1
  Memory1/1 -> Sum1/2
  Sum1/1 -> Saturation/1, Scope1/1, Memory1/1  "pid_integ"
  Sum6/1 -> Kp/1, dt/1, Memory/1, Sum2/1  "pid_error"
  1/dt/1 -> Kd/1
  Sum2/1 -> 1/dt/1
  dt/1 -> Sum1/1
  Kd/1 -> Sum5/3
  Kp/1 -> Sum5/1
  Sum5/1 -> Adjust/1
  Ki/1 -> Sum5/2
  Memory/1 -> Sum2/2  "pid_prevError"
  Setpoint/1 -> Sum6/1  "pid_desired"

== system PID_Controller_xynew_2018/old linear backup/Position_controller1/PID_Y2 ==
  Setpoint : Inport
  Measured : Inport  Port=2
  1/dt : Gain  Gain=100  OutMin=[-200]  OutMax=[200]
  Kd : Gain  Gain=0  OutMin=[-200]  OutMax=[200]
  Ki : Gain  Gain=-1  OutMin=[-200]  OutMax=[200]
  Kp : Gain  Gain=-15  OutMin=[-200]  OutMax=[200]
  Memory : Memory
  Memory1 : Memory
  Saturation : Saturate  UpperLimit=0.1  LowerLimit=-0.1
  Scope1 : Scope
  Scope2 : Scope
  Sum1 : Sum  Inputs=|++
  Sum2 : Sum  Inputs=|+-
  Sum5 : Sum  Inputs=+++
  Sum6 : Sum  Inputs=+-|
  dt : Gain  Gain=1/100  OutMin=[-200]  OutMax=[200]
  Adjust : Outport  VectorParamsAs1DForOutWhenUnconnected=on
  wires:
  Measured/1 -> Sum6/2
  Saturation/1 -> Ki/1, Scope2/1
  Memory1/1 -> Sum1/2
  Sum1/1 -> Saturation/1, Scope1/1, Memory1/1  "pid_integ"
  Sum6/1 -> Kp/1, dt/1, Memory/1, Sum2/1  "pid_error"
  1/dt/1 -> Kd/1
  Sum2/1 -> 1/dt/1
  dt/1 -> Sum1/1
  Kd/1 -> Sum5/3
  Kp/1 -> Sum5/1
  Sum5/1 -> Adjust/1
  Ki/1 -> Sum5/2
  Memory/1 -> Sum2/2  "pid_prevError"
  Setpoint/1 -> Sum6/1  "pid_desired"
